simulink model "TD2"  (R2024b)
settings: Solver=ode15s  StartTime=0.0  StopTime=1  RelTol=1e-3
InitFcn:
  | TD2_config
StartFcn:
  | TD2_config
values from neighbouring files (symbols this model uses):
  b = 8.5e-3    (= 0.0085)    [TD2_config.m]    (also in TD3_config.m)
  Cr = 0    [TD2_config.m]    (also in TD3_config.m)
  delay = 0.002    [TD3_config.m]
  J = 0.28    [TD2_config.m]    (also in TD3_config.m)
  K = Km    (= 0.5093)    [TD2_config.m]    (also in TD3_config.m)
  Ki = 50    [TD2_config.m]    (also in TD3_config.m = 40)
  Kp = 6    [TD2_config.m]    (also in TD3_config.m = 4)
  Kpos = 6    [TD2_config.m]    (also in TD3_config.m = 30)
  L = 1.6e-3    (= 0.0016)    [TD2_config.m]    (also in TD3_config.m)
  R = 0.13    [TD2_config.m]    (also in TD3_config.m)
  sampleTime = 0.01    [TD3_config.m]
libraries: simulink x1
settings Model: Creator=E306_PC2  LastModifiedBy=E306_PC2

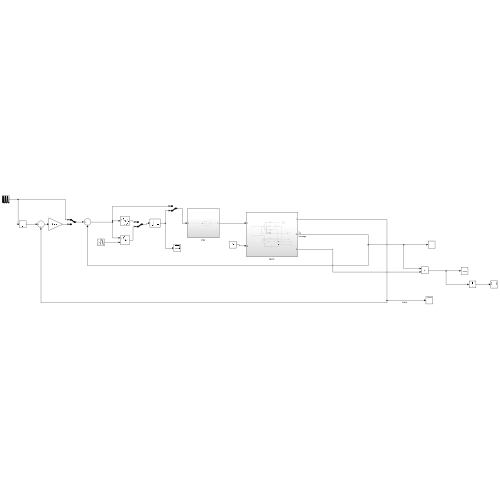
[thumbnail: Simulink's stored preview of the top-level diagram]
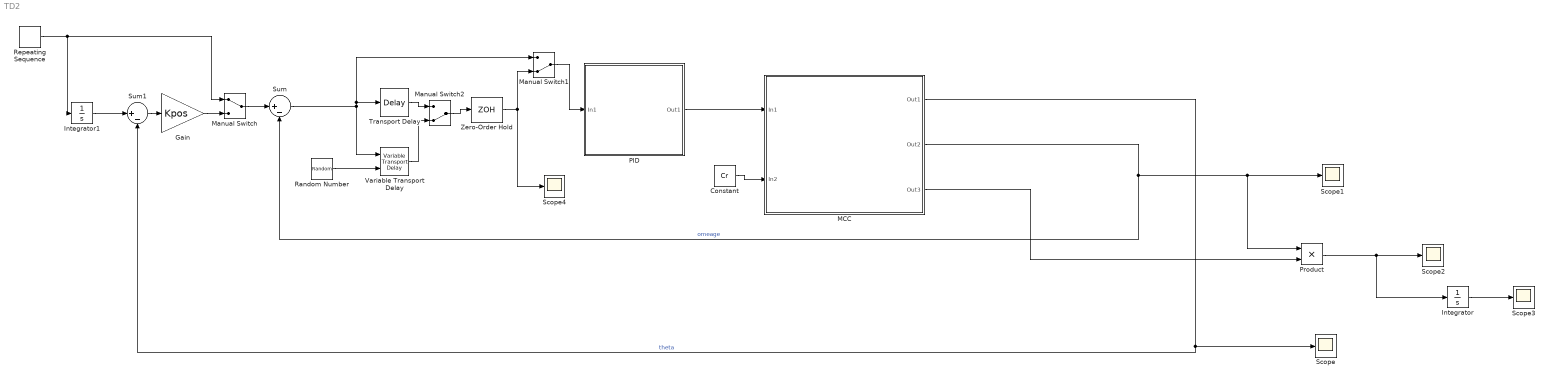
== system TD2 ==
  Constant : Constant  Value=Cr
  Gain : Gain  Gain=Kpos
  Integrator : Integrator
  Integrator1 : Integrator
  MCC : Subsystem
  Manual Switch : ManualSwitch
  Manual Switch1 : ManualSwitch  CurrentSetting=0
  Manual Switch2 : ManualSwitch  CurrentSetting=0
  PID : Subsystem
  Product : Product
  Random Number : RandomNumber  Mean=0.002  Variance=0.001  SampleTime=0.001
  Repeating Sequence : simulink/Sources/Repeating Sequence  rep_seq_t=[0 0.075 0.15 0.225 0.5]  rep_seq_y=[0 66.66 66.66 0 0 ]
  Scope{,1..4} (5 alike) : Scope
  Sum : Sum  Inputs=|+-
  Sum1 : Sum  Inputs=|+-
  Transport Delay : TransportDelay  DelayTime=delay
  Variable Transport Delay : VariableTransportDelay  VariableDelayType=Variable transport delay  MaximumDelay=10
  Zero-Order Hold : ZeroOrderHold  SampleTime=sampleTime
  wires:
  Constant/1 -> MCC/2(In2)
  MCC/1(Out1) -> Sum1/2, Scope/1  "theta"
  MCC/2(Out2) -> Sum/2, Product/1, Scope1/1  "omeage"
  Sum1/1 -> Gain/1
  Gain/1 -> Manual Switch/2
  Manual Switch/1 -> Sum/1
  MCC/3(Out3) -> Product/2
  Product/1 -> Integrator/1, Scope2/1
  Integrator/1 -> Scope3/1
  Repeating Sequence/1 -> Integrator1/1, Manual Switch/1
  Integrator1/1 -> Sum1/1
  Zero-Order Hold/1 -> Manual Switch1/2, Scope4/1
  Manual Switch1/1 -> PID/1(In1)
  Sum/1 -> Manual Switch1/1, Transport Delay/1, Variable Transport Delay/1
  PID/1(Out1) -> MCC/1(In1)
  Random Number/1 -> Variable Transport Delay/2
  Variable Transport Delay/1 -> Manual Switch2/2
  Transport Delay/1 -> Manual Switch2/1
  Manual Switch2/1 -> Zero-Order Hold/1

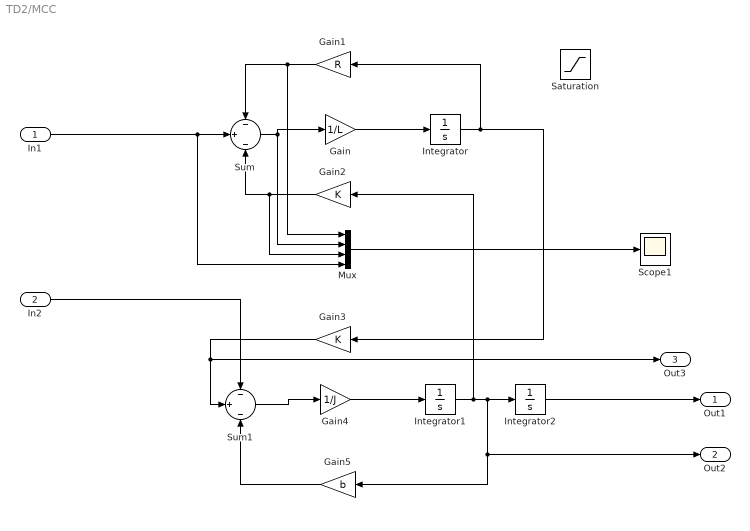
== system TD2/MCC ==
  In1 : Inport
  In2 : Inport  Port=2
  Gain : Gain  Gain=1/L
  Gain1 : Gain  Gain=R
  Gain2 : Gain  Gain=K
  Gain3 : Gain  Gain=K
  Gain4 : Gain  Gain=1/J
  Gain5 : Gain  Gain=b
  Integrator : Integrator
  Integrator1 : Integrator
  Integrator2 : Integrator
  Mux : Mux
  Saturation : Saturate  UpperLimit=80  LowerLimit=-70
  Scope1 : Scope
  Sum : Sum  Inputs=-|+|-
  Sum1 : Sum  Inputs=-|+|-
  Out1 : Outport
  Out2 : Outport  Port=2
  Out3 : Outport  Port=3
  wires:
  Integrator2/1 -> Out1/1
  Mux/1 -> Scope1/1
  Gain2/1 -> Mux/3, Sum/3
  Integrator1/1 -> Gain5/1, Out2/1, Integrator2/1, Gain2/1
  Gain1/1 -> Mux/1, Sum/1
  Gain5/1 -> Sum1/3
  In1/1 -> Mux/4, Sum/2
  Sum/1 -> Gain/1, Mux/2
  Gain4/1 -> Integrator1/1
  Gain/1 -> Integrator/1
  Gain3/1 -> Out3/1, Sum1/2
  Sum1/1 -> Gain4/1
  In2/1 -> Sum1/1
  Integrator/1 -> Gain3/1, Gain1/1

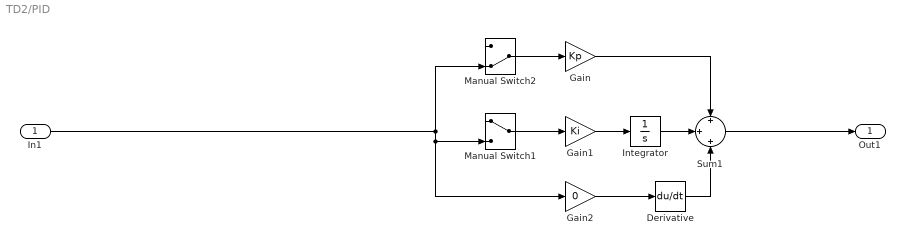
== system TD2/PID ==
  In1 : Inport
  Derivative : Derivative
  Gain : Gain  Gain=Kp
  Gain1 : Gain  Gain=Ki
  Gain2 : Gain  Gain=0
  Integrator : Integrator
  Manual Switch1 : ManualSwitch
  Manual Switch2 : ManualSwitch  CurrentSetting=0
  Sum1 : Sum  Inputs=+|+|+
  Out1 : Outport
  wires:
  Sum1/1 -> Out1/1
  Integrator/1 -> Sum1/2
  Gain1/1 -> Integrator/1
  Gain2/1 -> Derivative/1
  Derivative/1 -> Sum1/3
  Gain/1 -> Sum1/1
  In1/1 -> Manual Switch1/2, Gain2/1, Manual Switch2/2
  Manual Switch2/1 -> Gain/1
  Manual Switch1/1 -> Gain1/1
